simulink model "pi_simulation"  (R2023b)
settings: Solver=FixedStepAuto  StartTime=0.0  StopTime=sim_time  FixedStep=T_vz  RelTol=1e-3
values from neighbouring files (symbols this model uses):
  B_e = 0.05    [GA.m]    (also in exam.m = 0.001; grafs.m = gears(i); pi_GA.m; test.m = 0.001)
  B_m = 0.000080292    (= 8.0292e-05)    [GA.m]    (also in exam.m; pi_GA.m; test.m)
  B_z = 0.00020000    (= 0.0002)    [GA.m]    (also in exam.m; pi_GA.m; test.m)
  i_gear = 100    [GA.m]    (also in grafs.m = 20; pi_GA.m; test.m = 1)
  J_m = 0.00009    (= 9e-05)    [GA.m]    (also in exam.m; pi_GA.m; test.m)
  J_z = 0.00024943    [GA.m]    (also in exam.m; pi_GA.m; test.m)
  K_e = 0.5    [GA.m]    (also in exam.m = 0.01; grafs.m = gears(i); pi_GA.m; test.m = 0.01)
  Kd = 0.001    [test.m]
  Ki = 1.5    [test.m]
  Kp = 5    [test.m]
  M_m = 0.108    [GA.m]    (also in exam.m; pi_GA.m; test.m)
  M_z0m = 0.0052    [GA.m]    (also in exam.m; pi_GA.m; test.m)
  M_z0z = 0.0078    [GA.m]    (also in exam.m; pi_GA.m; test.m)
  N_el = 10000    [GA.m]    (also in exam.m; pi_GA.m; test.m)
  T_n = 0.001    [GA.m]    (also in exam.m; pi_GA.m; test.m)
  T_vz = 0.001    [GA.m]    (also in exam.m; pi_GA.m; test.m)
undefined symbols (not defined in the file or in its folder): DiscIntNeverNeededParam, param
libraries: slpidlib x6, simulink x3
settings Model: Creator=laptop  LastModifiedBy=maros-pc
settings SolverCC: ConsecutiveZCsStepRelTol=100000*128*eps  EnableFixedStepZeroCrossing=on  MaxZcPerStep=5
settings HardwareCC: ProdBitPerLong=64  ProdHWDeviceType=Intel->x86-64 (Linux 64)

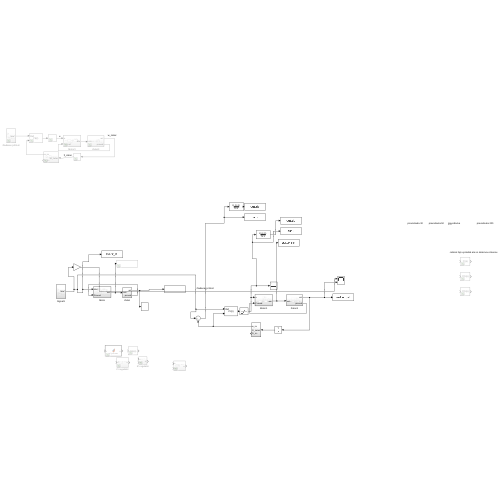
[thumbnail: Simulink's stored preview of the top-level diagram]
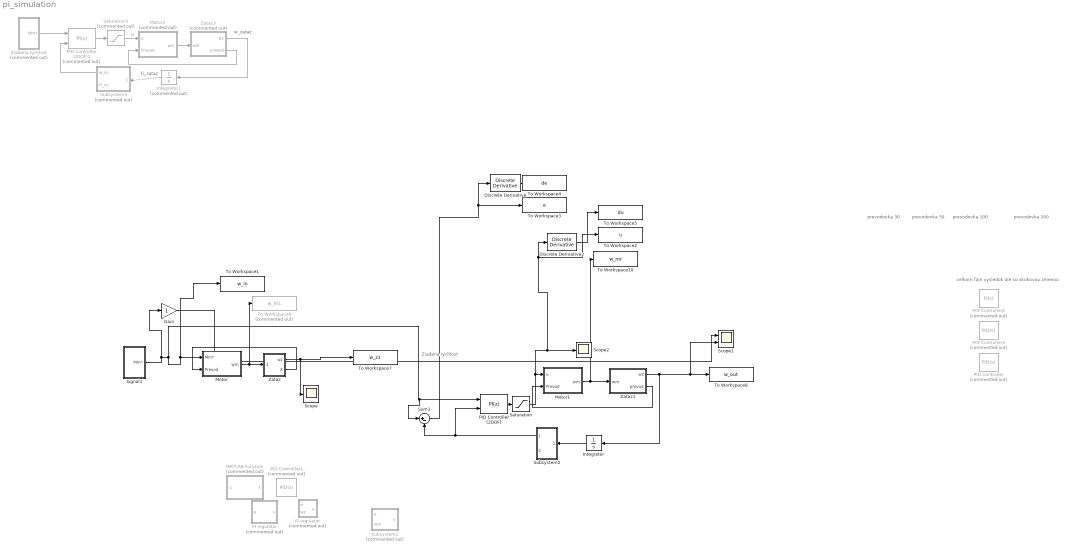
== system pi_simulation ==
  note: u
  note: w_zataz
  note: prevodovka 100
  note: celkom fajn vysledok ale so skokovou zmenou
  note: Ziadana rychlost
  note: prevodovka 200
  note: prevodovka 50
  note: prevodovka 30
  note: fi_zataz
  Discrete Derivative : simulink/Discrete/Discrete Derivative  gainval=1.0  ICPrevScaledInput=0.0  OutMin=[]  OutMax=[]  OutDataType=fixdt(1, 16)  OutScaling=2^-10  DoSatur=off
  Discrete Derivative2 : simulink/Discrete/Discrete Derivative  gainval=1.0  ICPrevScaledInput=0.0  OutMin=[]  OutMax=[]  OutDataType=fixdt(1, 16)  OutScaling=2^-10  DoSatur=off
  Gain : Gain
  IP regulator : Subsystem  Commented=on
  Integrator : Integrator
  Integrator1 : Integrator  Commented=on
  MATLAB Function : MATLAB Function  Commented=on  TreatAsAtomicUnit=on
  Motor : Subsystem
  Motor1 : Subsystem
  Motor3 : Subsystem  Commented=on
  PI regulator : Subsystem  Commented=on
  PID Controller : slpidlib/PID Controller  Commented=on  Controller=PID  Form=Parallel  TimeDomain=Continuous-time  UseExternalTs=off  SampleTime=-1  IntegratorMethod=Forward Euler  FilterMethod=Forward Euler  ControllerParametersSource=internal  P=param(1)  I=param(2)  UseKiTs=off  D=param(3)  N=param(4)  UseFilter=on  TunerSelectOption=Transfer Function Based (PID Tuner App)  InitialConditionSource=internal  InitialConditionForIntegrator=0  InitialConditionForFilter=0  DifferentiatorICPrevScaledInput=0  ExternalReset=none  TrackingMode=off  Kt=1  LimitOutput=off  SatLimitsSource=internal  UpperSaturationLimit=inf  LowerSaturationLimit=-inf  LinearizeAsGain=on  AntiWindupMode=none  Kb=1  LimitIntegrator=off  UpperIntegratorSaturationLimit=inf  LowerIntegratorSaturationLimit=-inf  POutMin=[]  POutMax=[]  IOutMin=[]  IOutMax=[]  DOutMin=[]  DOutMax=[]  NOutMin=[]  NOutMax=[]  SumOutMin=[]  SumOutMax=[]  SaturationOutMin=[]  SaturationOutMax=[]  PParamMin=[]  PParamMax=[]  IParamMin=[]  IParamMax=[]  DParamMin=[]  DParamMax=[]  NParamMin=[]  NParamMax=[]  KbParamMin=[]  KbParamMax=[]  KtParamMin=[]  KtParamMax=[]  KbOutMin=[]  KbOutMax=[]  KtOutMin=[]  KtOutMax=[]  IntegratorOutMin=[]  IntegratorOutMax=[]  FilterOutMin=[]  FilterOutMax=[]  SumI1OutMin=[]  SumI1OutMax=[]  SumI2OutMin=[]  SumI2OutMax=[]  SumI3OutMin=[]  SumI3OutMax=[]  SumI4OutMin=[]  SumI4OutMax=[]  SumDOutMin=[]  SumDOutMax=[]  DifferentiatorOutMin=[]  DifferentiatorOutMax=[]  FilterDiffOutCoefMin=[]  FilterDiffOutCoefMax=[]  ReciprocalOutMin=[]  ReciprocalOutMax=[]  SumDenOutMin=[]  SumDenOutMax=[]  SumNumOutMin=[]  SumNumOutMax=[]  DivideOutMin=[]  DivideOutMax=[]  UdiffTsProdOutMin=[]  UdiffTsProdOutMax=[]  NTsProdOutMin=[]  NTsProdOutMax=[]  UintegralTsProdOutMin=[]  UintegralTsProdOutMax=[]  UngainTsProdOutMin=[]  UngainTsProdOutMax=[]  ClampingZeroOutDataTypeStr=Inherit: Inherit via back propagation  ClampingZeroOutMin=[]  ClampingZeroOutMax=[]  FilterDenConstantOutDataTypeStr=Inherit: Inherit via back propagation  FilterDenConstantOutMin=[]  FilterDenConstantOutMax=[]  PCopyOutDataTypeStr=Inherit: Inherit via back propagation  PCopyOutMin=[]  PCopyOutMax=[]  NCopyOutDataTypeStr=Inherit: Inherit via back propagation  NCopyOutMin=[]  NCopyOutMax=[]  IntegratorContinuousStateAttributes=''  IntegratorStateMustResolveToSignalObject=off  IntegratorRTWStateStorageClass=Auto  FilterContinuousStateAttributes=''  FilterStateMustResolveToSignalObject=off  FilterRTWStateStorageClass=Auto  ParallelPVariant=InternalParameters  IdealPVariant=Disabled  IVariant=InternalParameters  DVariant=InternalParameters  IntegratorVariant=Continuous  SatVariant=Disabled  AWVariant=Passthrough  PCopyVariant=Disabled  TRVariant=Disabled  FdbkBlocksVariant=Forward  IdealPFdbkVariant=Disabled  SatFdbkVariant=Disabled  DerivativeFilterVariant=ContFilter  NVariant=InternalParameters  NCopyVariant=Disabled  FilterICVariant=InternalICsFilter  IntegratorICVariant=InternalICs  ExternalResetVariant=Disabled  TRSumVariant=Passthrough  SumFdbkVariant=Disabled  SumVariant=Sum_PID  TsampFilterVariant=InternalTs  TsampNgainVariant=Passthrough  TsampIntegralVariant=Disabled_SignalSpec  ExternalSaturationOutDataTypeStr=Inherit: Same as second input
  PID Controller (2DOF) : slpidlib/PID Controller (2DOF)  Controller=PI  Form=Parallel  TimeDomain=Discrete-time  UseExternalTs=off  SampleTime=T_vz  IntegratorMethod=Forward Euler  FilterMethod=Forward Euler  ControllerParametersSource=internal  P=param(1)  I=param(2)  UseKiTs=off  D=param(3)  N=param(4)  UseFilter=on  b=param(3)  c=param(6)  TunerSelectOption=Transfer Function Based (PID Tuner App)  InitialConditionSource=internal  InitialConditionForIntegrator=0  InitialConditionForFilter=0  DifferentiatorICPrevScaledInput=0  ExternalReset=none  TrackingMode=off  Kt=1  LimitOutput=off  SatLimitsSource=internal  UpperSaturationLimit=inf  LowerSaturationLimit=-inf  LinearizeAsGain=on  AntiWindupMode=none  Kb=1  LimitIntegrator=off  UpperIntegratorSaturationLimit=inf  LowerIntegratorSaturationLimit=-inf  POutMin=[]  POutMax=[]  IOutMin=[]  IOutMax=[]  DOutMin=[]  DOutMax=[]  NOutMin=[]  NOutMax=[]  bOutMin=[]  bOutMax=[]  cOutMin=[]  cOutMax=[]  SumOutMin=[]  SumOutMax=[]  SaturationOutMin=[]  SaturationOutMax=[]  PParamMin=[]  PParamMax=[]  IParamMin=[]  IParamMax=[]  DParamMin=[]  DParamMax=[]  NParamMin=[]  NParamMax=[]  bParamMin=[]  bParamMax=[]  cParamMin=[]  cParamMax=[]  KbParamMin=[]  KbParamMax=[]  KtParamMin=[]  KtParamMax=[]  KbOutMin=[]  KbOutMax=[]  KtOutMin=[]  KtOutMax=[]  IntegratorOutMin=[]  IntegratorOutMax=[]  FilterOutMin=[]  FilterOutMax=[]  SumI1OutMin=[]  SumI1OutMax=[]  SumI2OutMin=[]  SumI2OutMax=[]  SumI3OutMin=[]  SumI3OutMax=[]  SumI4OutMin=[]  SumI4OutMax=[]  SumDOutMin=[]  SumDOutMax=[]  Sum1OutMin=[]  Sum1OutMax=[]  Sum2OutMin=[]  Sum2OutMax=[]  Sum3OutMin=[]  Sum3OutMax=[]  DifferentiatorOutMin=[]  DifferentiatorOutMax=[]  FilterDiffOutCoefMin=[]  FilterDiffOutCoefMax=[]  ReciprocalOutMin=[]  ReciprocalOutMax=[]  SumDenOutMin=[]  SumDenOutMax=[]  SumNumOutMin=[]  SumNumOutMax=[]  DivideOutMin=[]  DivideOutMax=[]  UdiffTsProdOutMin=[]  UdiffTsProdOutMax=[]  NTsProdOutMin=[]  NTsProdOutMax=[]  UintegralTsProdOutMin=[]  UintegralTsProdOutMax=[]  UngainTsProdOutMin=[]  UngainTsProdOutMax=[]  ClampingZeroOutDataTypeStr=Inherit: Inherit via back propagation  ClampingZeroOutMin=[]  ClampingZeroOutMax=[]  FilterDenConstantOutDataTypeStr=Inherit: Inherit via back propagation  FilterDenConstantOutMin=[]  FilterDenConstantOutMax=[]  PCopyOutDataTypeStr=Inherit: Inherit via back propagation  PCopyOutMin=[]  PCopyOutMax=[]  NCopyOutDataTypeStr=Inherit: Inherit via back propagation  NCopyOutMin=[]  NCopyOutMax=[]  IntegratorContinuousStateAttributes=''  IntegratorStateMustResolveToSignalObject=off  IntegratorRTWStateStorageClass=Auto  FilterContinuousStateAttributes=''  FilterStateMustResolveToSignalObject=off  FilterRTWStateStorageClass=Auto  ParallelPVariant=InternalParameters  IdealPVariant=Disabled  IVariant=InternalParameters  DVariant=Disabled  bVariant=InternalParameters  cVariant=Disabled  IntegratorVariant=Discrete  SatVariant=Disabled  AWVariant=Passthrough  PCopyVariant=Disabled  TRVariant=Disabled  FdbkBlocksVariant=Forward  IdealPFdbkVariant=Disabled  SatFdbkVariant=Disabled  DerivativeFilterVariant=Disabled  NVariant=Disabled  NCopyVariant=Disabled_SignalSpec  FilterICVariant=Disabled  IntegratorICVariant=InternalICs  ExternalResetVariant=Disabled  TRSumVariant=Passthrough  SumFdbkVariant=Disabled  SumVariant=Sum_PI  TsampFilterVariant=InternalTs  TsampNgainVariant=Passthrough  TsampIntegralVariant=Disabled_SignalSpec  ExternalSaturationOutDataTypeStr=Inherit: Same as second input
  PID Controller (2DOF)1 : slpidlib/PID Controller (2DOF)  Commented=on  Controller=PI  Form=Parallel  TimeDomain=Discrete-time  UseExternalTs=off  SampleTime=T_vz  IntegratorMethod=Forward Euler  FilterMethod=Forward Euler  ControllerParametersSource=internal  P=param(1)  I=param(2)  UseKiTs=off  D=param(3)  N=param(4)  UseFilter=on  b=param(3)  c=param(6)  TunerSelectOption=Transfer Function Based (PID Tuner App)  InitialConditionSource=internal  InitialConditionForIntegrator=0  InitialConditionForFilter=0  DifferentiatorICPrevScaledInput=0  ExternalReset=none  TrackingMode=off  Kt=1  LimitOutput=off  SatLimitsSource=internal  UpperSaturationLimit=inf  LowerSaturationLimit=-inf  LinearizeAsGain=on  AntiWindupMode=none  Kb=1  LimitIntegrator=off  UpperIntegratorSaturationLimit=inf  LowerIntegratorSaturationLimit=-inf  POutMin=[]  POutMax=[]  IOutMin=[]  IOutMax=[]  DOutMin=[]  DOutMax=[]  NOutMin=[]  NOutMax=[]  bOutMin=[]  bOutMax=[]  cOutMin=[]  cOutMax=[]  SumOutMin=[]  SumOutMax=[]  SaturationOutMin=[]  SaturationOutMax=[]  PParamMin=[]  PParamMax=[]  IParamMin=[]  IParamMax=[]  DParamMin=[]  DParamMax=[]  NParamMin=[]  NParamMax=[]  bParamMin=[]  bParamMax=[]  cParamMin=[]  cParamMax=[]  KbParamMin=[]  KbParamMax=[]  KtParamMin=[]  KtParamMax=[]  KbOutMin=[]  KbOutMax=[]  KtOutMin=[]  KtOutMax=[]  IntegratorOutMin=[]  IntegratorOutMax=[]  FilterOutMin=[]  FilterOutMax=[]  SumI1OutMin=[]  SumI1OutMax=[]  SumI2OutMin=[]  SumI2OutMax=[]  SumI3OutMin=[]  SumI3OutMax=[]  SumI4OutMin=[]  SumI4OutMax=[]  SumDOutMin=[]  SumDOutMax=[]  Sum1OutMin=[]  Sum1OutMax=[]  Sum2OutMin=[]  Sum2OutMax=[]  Sum3OutMin=[]  Sum3OutMax=[]  DifferentiatorOutMin=[]  DifferentiatorOutMax=[]  FilterDiffOutCoefMin=[]  FilterDiffOutCoefMax=[]  ReciprocalOutMin=[]  ReciprocalOutMax=[]  SumDenOutMin=[]  SumDenOutMax=[]  SumNumOutMin=[]  SumNumOutMax=[]  DivideOutMin=[]  DivideOutMax=[]  UdiffTsProdOutMin=[]  UdiffTsProdOutMax=[]  NTsProdOutMin=[]  NTsProdOutMax=[]  UintegralTsProdOutMin=[]  UintegralTsProdOutMax=[]  UngainTsProdOutMin=[]  UngainTsProdOutMax=[]  ClampingZeroOutDataTypeStr=Inherit: Inherit via back propagation  ClampingZeroOutMin=[]  ClampingZeroOutMax=[]  FilterDenConstantOutDataTypeStr=Inherit: Inherit via back propagation  FilterDenConstantOutMin=[]  FilterDenConstantOutMax=[]  PCopyOutDataTypeStr=Inherit: Inherit via back propagation  PCopyOutMin=[]  PCopyOutMax=[]  NCopyOutDataTypeStr=Inherit: Inherit via back propagation  NCopyOutMin=[]  NCopyOutMax=[]  IntegratorContinuousStateAttributes=''  IntegratorStateMustResolveToSignalObject=off  IntegratorRTWStateStorageClass=Auto  FilterContinuousStateAttributes=''  FilterStateMustResolveToSignalObject=off  FilterRTWStateStorageClass=Auto  ParallelPVariant=InternalParameters  IdealPVariant=Disabled  IVariant=InternalParameters  DVariant=Disabled  bVariant=InternalParameters  cVariant=Disabled  IntegratorVariant=Discrete  SatVariant=Disabled  AWVariant=Passthrough  PCopyVariant=Disabled  TRVariant=Disabled  FdbkBlocksVariant=Forward  IdealPFdbkVariant=Disabled  SatFdbkVariant=Disabled  DerivativeFilterVariant=Disabled  NVariant=Disabled  NCopyVariant=Disabled_SignalSpec  FilterICVariant=Disabled  IntegratorICVariant=InternalICs  ExternalResetVariant=Disabled  TRSumVariant=Passthrough  SumFdbkVariant=Disabled  SumVariant=Sum_PI  TsampFilterVariant=InternalTs  TsampNgainVariant=Passthrough  TsampIntegralVariant=Disabled_SignalSpec  ExternalSaturationOutDataTypeStr=Inherit: Same as second input
  PID Controller1 : slpidlib/PID Controller  Commented=on  Controller=PID  Form=Parallel  TimeDomain=Continuous-time  UseExternalTs=off  SampleTime=-1  IntegratorMethod=Forward Euler  FilterMethod=Forward Euler  ControllerParametersSource=internal  P=0.00289759486685387  I=0.00379715777918526  UseKiTs=off  D=-0.00216183829362266  N=1.34033839413506  UseFilter=on  TunerSelectOption=Transfer Function Based (PID Tuner App)  InitialConditionSource=internal  InitialConditionForIntegrator=0  InitialConditionForFilter=0  DifferentiatorICPrevScaledInput=0  ExternalReset=none  TrackingMode=off  Kt=1  LimitOutput=off  SatLimitsSource=internal  UpperSaturationLimit=inf  LowerSaturationLimit=-inf  LinearizeAsGain=on  AntiWindupMode=none  Kb=1  LimitIntegrator=off  UpperIntegratorSaturationLimit=inf  LowerIntegratorSaturationLimit=-inf  POutMin=[]  POutMax=[]  IOutMin=[]  IOutMax=[]  DOutMin=[]  DOutMax=[]  NOutMin=[]  NOutMax=[]  SumOutMin=[]  SumOutMax=[]  SaturationOutMin=[]  SaturationOutMax=[]  PParamMin=[]  PParamMax=[]  IParamMin=[]  IParamMax=[]  DParamMin=[]  DParamMax=[]  NParamMin=[]  NParamMax=[]  KbParamMin=[]  KbParamMax=[]  KtParamMin=[]  KtParamMax=[]  KbOutMin=[]  KbOutMax=[]  KtOutMin=[]  KtOutMax=[]  IntegratorOutMin=[]  IntegratorOutMax=[]  FilterOutMin=[]  FilterOutMax=[]  SumI1OutMin=[]  SumI1OutMax=[]  SumI2OutMin=[]  SumI2OutMax=[]  SumI3OutMin=[]  SumI3OutMax=[]  SumI4OutMin=[]  SumI4OutMax=[]  SumDOutMin=[]  SumDOutMax=[]  DifferentiatorOutMin=[]  DifferentiatorOutMax=[]  FilterDiffOutCoefMin=[]  FilterDiffOutCoefMax=[]  ReciprocalOutMin=[]  ReciprocalOutMax=[]  SumDenOutMin=[]  SumDenOutMax=[]  SumNumOutMin=[]  SumNumOutMax=[]  DivideOutMin=[]  DivideOutMax=[]  UdiffTsProdOutMin=[]  UdiffTsProdOutMax=[]  NTsProdOutMin=[]  NTsProdOutMax=[]  UintegralTsProdOutMin=[]  UintegralTsProdOutMax=[]  UngainTsProdOutMin=[]  UngainTsProdOutMax=[]  ClampingZeroOutDataTypeStr=Inherit: Inherit via back propagation  ClampingZeroOutMin=[]  ClampingZeroOutMax=[]  FilterDenConstantOutDataTypeStr=Inherit: Inherit via back propagation  FilterDenConstantOutMin=[]  FilterDenConstantOutMax=[]  PCopyOutDataTypeStr=Inherit: Inherit via back propagation  PCopyOutMin=[]  PCopyOutMax=[]  NCopyOutDataTypeStr=Inherit: Inherit via back propagation  NCopyOutMin=[]  NCopyOutMax=[]  IntegratorContinuousStateAttributes=''  IntegratorStateMustResolveToSignalObject=off  IntegratorRTWStateStorageClass=Auto  FilterContinuousStateAttributes=''  FilterStateMustResolveToSignalObject=off  FilterRTWStateStorageClass=Auto  ParallelPVariant=InternalParameters  IdealPVariant=Disabled  IVariant=InternalParameters  DVariant=InternalParameters  IntegratorVariant=Continuous  SatVariant=Disabled  AWVariant=Passthrough  PCopyVariant=Disabled  TRVariant=Disabled  FdbkBlocksVariant=Forward  IdealPFdbkVariant=Disabled  SatFdbkVariant=Disabled  DerivativeFilterVariant=ContFilter  NVariant=InternalParameters  NCopyVariant=Disabled  FilterICVariant=InternalICsFilter  IntegratorICVariant=InternalICs  ExternalResetVariant=Disabled  TRSumVariant=Passthrough  SumFdbkVariant=Disabled  SumVariant=Sum_PID  TsampFilterVariant=InternalTs  TsampNgainVariant=Passthrough  TsampIntegralVariant=Disabled_SignalSpec  ExternalSaturationOutDataTypeStr=Inherit: Same as second input
  PID Controller2 : slpidlib/PID Controller  Commented=on  Controller=PI  Form=Parallel  TimeDomain=Continuous-time  UseExternalTs=off  SampleTime=-1  IntegratorMethod=Forward Euler  FilterMethod=Forward Euler  ControllerParametersSource=internal  P=0.0039717054355857  I=0.00555616938335056  UseKiTs=off  D=0  N=100  UseFilter=on  TunerSelectOption=Transfer Function Based (PID Tuner App)  InitialConditionSource=internal  InitialConditionForIntegrator=0  InitialConditionForFilter=0  DifferentiatorICPrevScaledInput=0  ExternalReset=none  TrackingMode=off  Kt=1  LimitOutput=off  SatLimitsSource=internal  UpperSaturationLimit=inf  LowerSaturationLimit=-inf  LinearizeAsGain=on  AntiWindupMode=none  Kb=1  LimitIntegrator=off  UpperIntegratorSaturationLimit=inf  LowerIntegratorSaturationLimit=-inf  POutMin=[]  POutMax=[]  IOutMin=[]  IOutMax=[]  DOutMin=[]  DOutMax=[]  NOutMin=[]  NOutMax=[]  SumOutMin=[]  SumOutMax=[]  SaturationOutMin=[]  SaturationOutMax=[]  PParamMin=[]  PParamMax=[]  IParamMin=[]  IParamMax=[]  DParamMin=[]  DParamMax=[]  NParamMin=[]  NParamMax=[]  KbParamMin=[]  KbParamMax=[]  KtParamMin=[]  KtParamMax=[]  KbOutMin=[]  KbOutMax=[]  KtOutMin=[]  KtOutMax=[]  IntegratorOutMin=[]  IntegratorOutMax=[]  FilterOutMin=[]  FilterOutMax=[]  SumI1OutMin=[]  SumI1OutMax=[]  SumI2OutMin=[]  SumI2OutMax=[]  SumI3OutMin=[]  SumI3OutMax=[]  SumI4OutMin=[]  SumI4OutMax=[]  SumDOutMin=[]  SumDOutMax=[]  DifferentiatorOutMin=[]  DifferentiatorOutMax=[]  FilterDiffOutCoefMin=[]  FilterDiffOutCoefMax=[]  ReciprocalOutMin=[]  ReciprocalOutMax=[]  SumDenOutMin=[]  SumDenOutMax=[]  SumNumOutMin=[]  SumNumOutMax=[]  DivideOutMin=[]  DivideOutMax=[]  UdiffTsProdOutMin=[]  UdiffTsProdOutMax=[]  NTsProdOutMin=[]  NTsProdOutMax=[]  UintegralTsProdOutMin=[]  UintegralTsProdOutMax=[]  UngainTsProdOutMin=[]  UngainTsProdOutMax=[]  ClampingZeroOutDataTypeStr=Inherit: Inherit via back propagation  ClampingZeroOutMin=[]  ClampingZeroOutMax=[]  FilterDenConstantOutDataTypeStr=Inherit: Inherit via back propagation  FilterDenConstantOutMin=[]  FilterDenConstantOutMax=[]  PCopyOutDataTypeStr=Inherit: Inherit via back propagation  PCopyOutMin=[]  PCopyOutMax=[]  NCopyOutDataTypeStr=Inherit: Inherit via back propagation  NCopyOutMin=[]  NCopyOutMax=[]  IntegratorContinuousStateAttributes=''  IntegratorStateMustResolveToSignalObject=off  IntegratorRTWStateStorageClass=Auto  FilterContinuousStateAttributes=''  FilterStateMustResolveToSignalObject=off  FilterRTWStateStorageClass=Auto  ParallelPVariant=InternalParameters  IdealPVariant=Disabled  IVariant=InternalParameters  DVariant=Disabled  IntegratorVariant=Continuous  SatVariant=Disabled  AWVariant=Passthrough  PCopyVariant=Disabled  TRVariant=Disabled  FdbkBlocksVariant=Forward  IdealPFdbkVariant=Disabled  SatFdbkVariant=Disabled  DerivativeFilterVariant=Disabled  NVariant=Disabled  NCopyVariant=Disabled_SignalSpec  FilterICVariant=Disabled  IntegratorICVariant=InternalICs  ExternalResetVariant=Disabled  TRSumVariant=Passthrough  SumFdbkVariant=Disabled  SumVariant=Sum_PI  TsampFilterVariant=InternalTs  TsampNgainVariant=Passthrough  TsampIntegralVariant=Disabled_SignalSpec  ExternalSaturationOutDataTypeStr=Inherit: Same as second input
  PID Controller3 : slpidlib/PID Controller  Commented=on  Controller=PID  Form=Parallel  TimeDomain=Continuous-time  UseExternalTs=off  SampleTime=-1  IntegratorMethod=Forward Euler  FilterMethod=Forward Euler  ControllerParametersSource=internal  P=0.00146819518976187  I=0.0028749942576144  UseKiTs=off  D=-0.001808078912925  N=0.812019419764548  UseFilter=on  TunerSelectOption=Transfer Function Based (PID Tuner App)  InitialConditionSource=internal  InitialConditionForIntegrator=0  InitialConditionForFilter=0  DifferentiatorICPrevScaledInput=0  ExternalReset=none  TrackingMode=off  Kt=1  LimitOutput=off  SatLimitsSource=internal  UpperSaturationLimit=inf  LowerSaturationLimit=-inf  LinearizeAsGain=on  AntiWindupMode=none  Kb=1  LimitIntegrator=off  UpperIntegratorSaturationLimit=inf  LowerIntegratorSaturationLimit=-inf  POutMin=[]  POutMax=[]  IOutMin=[]  IOutMax=[]  DOutMin=[]  DOutMax=[]  NOutMin=[]  NOutMax=[]  SumOutMin=[]  SumOutMax=[]  SaturationOutMin=[]  SaturationOutMax=[]  PParamMin=[]  PParamMax=[]  IParamMin=[]  IParamMax=[]  DParamMin=[]  DParamMax=[]  NParamMin=[]  NParamMax=[]  KbParamMin=[]  KbParamMax=[]  KtParamMin=[]  KtParamMax=[]  KbOutMin=[]  KbOutMax=[]  KtOutMin=[]  KtOutMax=[]  IntegratorOutMin=[]  IntegratorOutMax=[]  FilterOutMin=[]  FilterOutMax=[]  SumI1OutMin=[]  SumI1OutMax=[]  SumI2OutMin=[]  SumI2OutMax=[]  SumI3OutMin=[]  SumI3OutMax=[]  SumI4OutMin=[]  SumI4OutMax=[]  SumDOutMin=[]  SumDOutMax=[]  DifferentiatorOutMin=[]  DifferentiatorOutMax=[]  FilterDiffOutCoefMin=[]  FilterDiffOutCoefMax=[]  ReciprocalOutMin=[]  ReciprocalOutMax=[]  SumDenOutMin=[]  SumDenOutMax=[]  SumNumOutMin=[]  SumNumOutMax=[]  DivideOutMin=[]  DivideOutMax=[]  UdiffTsProdOutMin=[]  UdiffTsProdOutMax=[]  NTsProdOutMin=[]  NTsProdOutMax=[]  UintegralTsProdOutMin=[]  UintegralTsProdOutMax=[]  UngainTsProdOutMin=[]  UngainTsProdOutMax=[]  ClampingZeroOutDataTypeStr=Inherit: Inherit via back propagation  ClampingZeroOutMin=[]  ClampingZeroOutMax=[]  FilterDenConstantOutDataTypeStr=Inherit: Inherit via back propagation  FilterDenConstantOutMin=[]  FilterDenConstantOutMax=[]  PCopyOutDataTypeStr=Inherit: Inherit via back propagation  PCopyOutMin=[]  PCopyOutMax=[]  NCopyOutDataTypeStr=Inherit: Inherit via back propagation  NCopyOutMin=[]  NCopyOutMax=[]  IntegratorContinuousStateAttributes=''  IntegratorStateMustResolveToSignalObject=off  IntegratorRTWStateStorageClass=Auto  FilterContinuousStateAttributes=''  FilterStateMustResolveToSignalObject=off  FilterRTWStateStorageClass=Auto  ParallelPVariant=InternalParameters  IdealPVariant=Disabled  IVariant=InternalParameters  DVariant=InternalParameters  IntegratorVariant=Continuous  SatVariant=Disabled  AWVariant=Passthrough  PCopyVariant=Disabled  TRVariant=Disabled  FdbkBlocksVariant=Forward  IdealPFdbkVariant=Disabled  SatFdbkVariant=Disabled  DerivativeFilterVariant=ContFilter  NVariant=InternalParameters  NCopyVariant=Disabled  FilterICVariant=InternalICsFilter  IntegratorICVariant=InternalICs  ExternalResetVariant=Disabled  TRSumVariant=Passthrough  SumFdbkVariant=Disabled  SumVariant=Sum_PID  TsampFilterVariant=InternalTs  TsampNgainVariant=Passthrough  TsampIntegralVariant=Disabled_SignalSpec  ExternalSaturationOutDataTypeStr=Inherit: Same as second input
  Saturation : Saturate  UpperLimit=M_m*0.75  LowerLimit=-M_m*0.75
  Saturation1 : Saturate  Commented=on  UpperLimit=M_m*0.75  LowerLimit=-M_m*0.75
  Scope : Scope
  Scope1 : Scope  NumInputPorts=2
  Scope2 : Scope
  Signal1 : Subsystem
  Subsystem1 : Subsystem  Commented=on
  Subsystem2 : Subsystem
  Subsystem3 : Subsystem  Commented=on
  Sum1 : Sum  Inputs=|+-
  To Workspace1 : ToWorkspace  VariableName=w_in  SaveFormat=Timeseries  SampleTime=-1
  To Workspace10 : ToWorkspace  VariableName=w_mr  SaveFormat=Timeseries  SampleTime=-1
  To Workspace2 : ToWorkspace  VariableName=u  SaveFormat=Timeseries  SampleTime=-1
  To Workspace3 : ToWorkspace  VariableName=e  SaveFormat=Timeseries  SampleTime=-1
  To Workspace4 : ToWorkspace  VariableName=de  SaveFormat=Timeseries  SampleTime=-1
  To Workspace5 : ToWorkspace  VariableName=du  SaveFormat=Timeseries  SampleTime=-1
  To Workspace7 : ToWorkspace  VariableName=w_z1  SaveFormat=Timeseries  SampleTime=-1
  To Workspace8 : ToWorkspace  VariableName=w_out  SaveFormat=Timeseries  SampleTime=-1
  To Workspace9 : ToWorkspace  Commented=on  VariableName=w_m1  SaveFormat=Timeseries  SampleTime=-1
  Zataz : Subsystem
  Zataz1 : Subsystem
  Zataz3 : Subsystem  Commented=on
  "Ziadana rychlost " : Subsystem  Commented=on
  wires:
  Motor/1(wm) -> To Workspace9/1, Zataz/1(wm)
  Zataz/1(wz) -> Scope/1, To Workspace7/1
  Zataz/2(prevod) -> Motor/2(Prevod)
  Zataz1/2(prevod) -> Motor1/2(Prevod)
  Zataz1/1(wz) -> Integrator/1, Scope1/2, To Workspace8/1
  Motor1/1(wm) -> To Workspace10/1, Zataz1/1(wm)
  Integrator/1 -> Subsystem2/1(Fi_zataz)
  Subsystem2/1(w_irc) -> Sum1/2, PID Controller (2DOF)/2
  Signal1/1(Mm*) -> Gain/1, Sum1/1, PID Controller (2DOF)/1, To Workspace1/1, Motor/1(Mm*)
  Discrete Derivative/1 -> To Workspace4/1
  Discrete Derivative2/1 -> To Workspace5/1
  Sum1/1 -> Discrete Derivative/1, To Workspace3/1
  Saturation/1 -> To Workspace2/1, Discrete Derivative2/1, Scope2/1, Motor1/1(u)
  PID Controller (2DOF)/1 -> Saturation/1
  Gain/1 -> Scope1/1
  PID Controller (2DOF)1/1 -> Saturation1/1
  Motor3/1(wm) -> Zataz3/1(wm)
  Subsystem3/1(w_irc) -> PID Controller (2DOF)1/2
  Zataz3/2(prevod) -> Motor3/2(Prevod)
  Saturation1/1 -> Motor3/1(u)
  Integrator1/1 -> Subsystem3/1(Fi_zataz)
  Zataz3/1(wz) -> Integrator1/1
  "Ziadana rychlost "/1(Mm*) -> PID Controller (2DOF)1/1

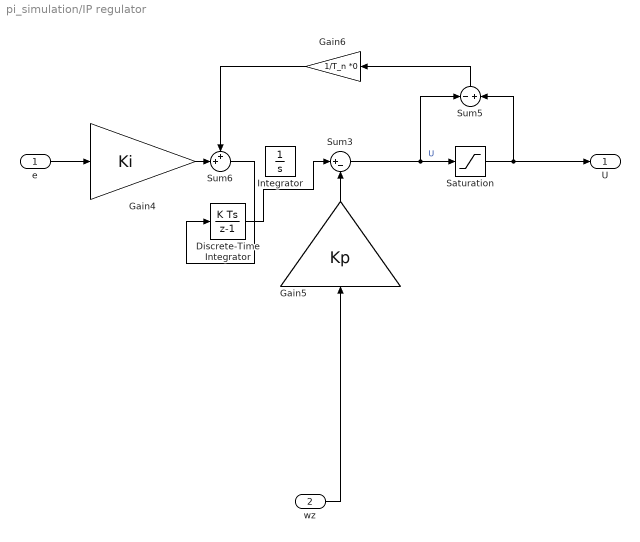
== system pi_simulation/IP regulator ==
  e : Inport
  wz : Inport  Port=2
  Discrete-Time Integrator : DiscreteIntegrator  SampleTime=-1  ICPrevOutput=DiscIntNeverNeededParam  ICPrevScaledInput=DiscIntNeverNeededParam
  Gain4 : Gain  Gain=Ki
  Gain5 : Gain  Gain=Kp
  Gain6 : Gain  Gain=1/T_n *0
  Integrator : Integrator
  Saturation : Saturate  UpperLimit=M_m*0.75  LowerLimit=-M_m*0.75
  Sum3 : Sum  Inputs=|+-
  Sum5 : Sum  Inputs=-+
  Sum6 : Sum  Inputs=++|
  U : Outport
  wires:
  Gain5/1 -> Sum3/2
  Gain4/1 -> Sum6/2
  Saturation/1 -> U/1, Sum5/2  "U"
  Sum5/1 -> Gain6/1
  Discrete-Time Integrator/1 -> Sum3/1
  Gain6/1 -> Sum6/1
  Sum3/1 -> Sum5/1, Saturation/1
  Sum6/1 -> Discrete-Time Integrator/1
  wz/1 -> Gain5/1
  e/1 -> Gain4/1

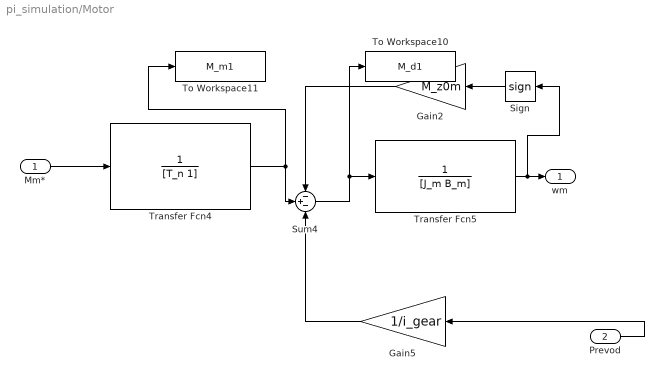
== system pi_simulation/Motor ==
  Mm* : Inport
  Prevod : Inport  Port=2
  Gain2 : Gain  Gain=M_z0m
  Gain5 : Gain  Gain=1/i_gear
  Sign : Signum
  Sum4 : Sum  Inputs=-+-
  To Workspace10 : ToWorkspace  VariableName=M_d1  SaveFormat=Timeseries  SampleTime=-1
  To Workspace11 : ToWorkspace  VariableName=M_m1  SaveFormat=Timeseries  SampleTime=-1
  Transfer Fcn4 : TransferFcn  Denominator=[T_n 1]
  Transfer Fcn5 : TransferFcn  Denominator=[J_m B_m]
  wm : Outport
  wires:
  Gain5/1 -> Sum4/3
  Sum4/1 -> To Workspace10/1, Transfer Fcn5/1
  Transfer Fcn4/1 -> Sum4/2, To Workspace11/1
  Mm*/1 -> Transfer Fcn4/1
  Prevod/1 -> Gain5/1
  Sign/1 -> Gain2/1
  Gain2/1 -> Sum4/1
  Transfer Fcn5/1 -> Sign/1, wm/1

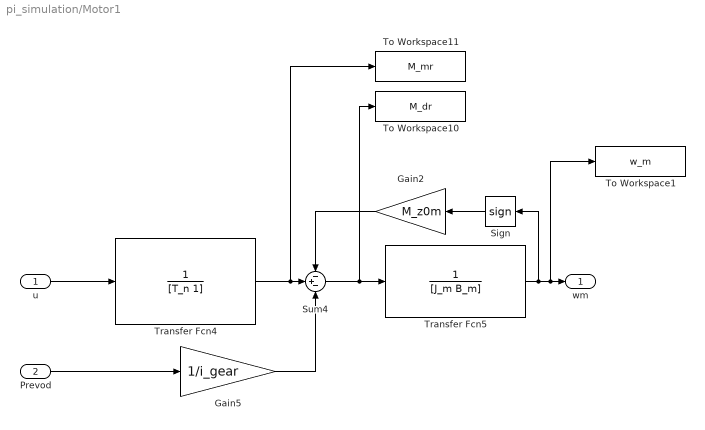
== system pi_simulation/Motor1 ==
  u : Inport
  Prevod : Inport  Port=2
  Gain2 : Gain  Gain=M_z0m
  Gain5 : Gain  Gain=1/i_gear
  Sign : Signum
  Sum4 : Sum  Inputs=-+-
  To Workspace1 : ToWorkspace  VariableName=w_m  SaveFormat=Timeseries  SampleTime=-1
  To Workspace10 : ToWorkspace  VariableName=M_dr  SaveFormat=Timeseries  SampleTime=-1
  To Workspace11 : ToWorkspace  VariableName=M_mr  SaveFormat=Timeseries  SampleTime=-1
  Transfer Fcn4 : TransferFcn  Denominator=[T_n 1]
  Transfer Fcn5 : TransferFcn  Denominator=[J_m B_m]
  wm : Outport
  wires:
  Gain5/1 -> Sum4/3
  Sum4/1 -> To Workspace10/1, Transfer Fcn5/1
  Transfer Fcn4/1 -> To Workspace11/1, Sum4/2
  u/1 -> Transfer Fcn4/1
  Prevod/1 -> Gain5/1
  Gain2/1 -> Sum4/1
  Transfer Fcn5/1 -> Sign/1, To Workspace1/1, wm/1
  Sign/1 -> Gain2/1

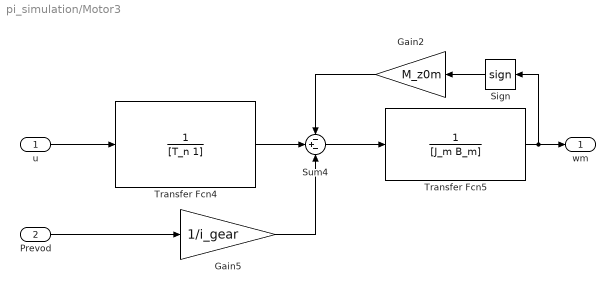
== system pi_simulation/Motor3 ==
  u : Inport
  Prevod : Inport  Port=2
  Gain2 : Gain  Gain=M_z0m
  Gain5 : Gain  Gain=1/i_gear
  Sign : Signum
  Sum4 : Sum  Inputs=-+-
  Transfer Fcn4 : TransferFcn  Denominator=[T_n 1]
  Transfer Fcn5 : TransferFcn  Denominator=[J_m B_m]
  wm : Outport
  wires:
  Gain5/1 -> Sum4/3
  Sum4/1 -> Transfer Fcn5/1
  Transfer Fcn4/1 -> Sum4/2
  u/1 -> Transfer Fcn4/1
  Prevod/1 -> Gain5/1
  Gain2/1 -> Sum4/1
  Transfer Fcn5/1 -> Sign/1, wm/1
  Sign/1 -> Gain2/1

== system pi_simulation/PI regulator ==
  e : Inport
  Discrete-Time Integrator : DiscreteIntegrator  SampleTime=T_vz  ICPrevOutput=DiscIntNeverNeededParam  ICPrevScaledInput=DiscIntNeverNeededParam
  Gain1 : Gain  Gain=Kp
  Gain2 : Gain  Gain=Ki
  Saturation : Saturate  UpperLimit=M_m*0.75  LowerLimit=-M_m*0.75
  Sum1 : Sum  Inputs=|++
  u : Outport
  wires:
  Gain1/1 -> Sum1/1
  Discrete-Time Integrator/1 -> Sum1/2
  Sum1/1 -> Saturation/1
  Gain2/1 -> Discrete-Time Integrator/1
  e/1 -> Gain2/1, Gain1/1
  Saturation/1 -> u/1  "U"

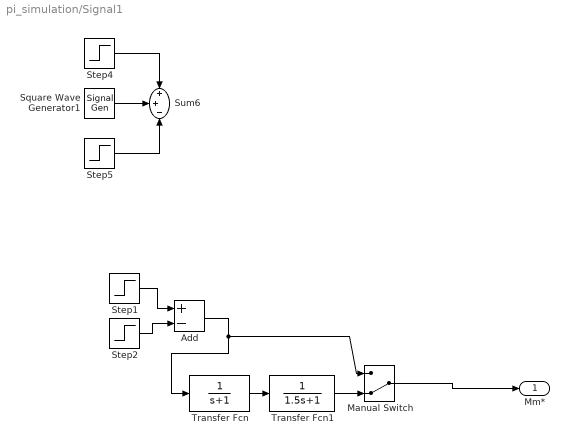
== system pi_simulation/Signal1 ==
  Add : Sum  Inputs=+-
  Manual Switch : ManualSwitch  CurrentSetting=0
  Square Wave Generator1 : SignalGenerator  Amplitude=0.8  Frequency=2
  Step1 : Step  After=pi/2  SampleTime=0
  Step2 : Step  Time=10  After=pi/2  SampleTime=0
  Step4 : Step  SampleTime=0
  Step5 : Step  Time=2  SampleTime=0
  Sum6 : Sum  Inputs=++-
  Transfer Fcn : TransferFcn  Denominator=[1 1]
  Transfer Fcn1 : TransferFcn  Denominator=[1.5 1]
  Mm* : Outport
  wires:
  Step4/1 -> Sum6/1
  Square Wave Generator1/1 -> Sum6/2
  Step5/1 -> Sum6/3
  Step1/1 -> Add/1
  Step2/1 -> Add/2
  Transfer Fcn/1 -> Transfer Fcn1/1
  Transfer Fcn1/1 -> Manual Switch/2
  Manual Switch/1 -> Mm*/1
  Add/1 -> Manual Switch/1, Transfer Fcn/1

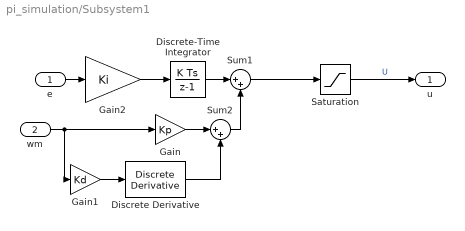
== system pi_simulation/Subsystem1 ==
  e : Inport
  wm : Inport  Port=2
  Discrete Derivative : simulink/Discrete/Discrete Derivative  gainval=1.0  ICPrevScaledInput=0.0  OutMin=[]  OutMax=[]  OutDataType=fixdt(1, 16)  OutScaling=2^-10  DoSatur=off
  Discrete-Time Integrator : DiscreteIntegrator  SampleTime=T_vz  ICPrevOutput=DiscIntNeverNeededParam  ICPrevScaledInput=DiscIntNeverNeededParam
  Gain : Gain  Gain=Kp
  Gain1 : Gain  Gain=Kd
  Gain2 : Gain  Gain=Ki
  Saturation : Saturate  UpperLimit=M_m*0.75  LowerLimit=-M_m*0.75
  Sum1 : Sum  Inputs=|++
  Sum2 : Sum  Inputs=|++
  u : Outport
  wires:
  Discrete-Time Integrator/1 -> Sum1/1
  Sum1/1 -> Saturation/1
  Gain2/1 -> Discrete-Time Integrator/1
  e/1 -> Gain2/1
  Saturation/1 -> u/1  "U"
  Gain1/1 -> Discrete Derivative/1
  Gain/1 -> Sum2/1
  Discrete Derivative/1 -> Sum2/2
  Sum2/1 -> Sum1/2
  wm/1 -> Gain1/1, Gain/1

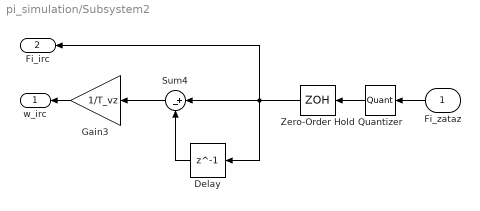
== system pi_simulation/Subsystem2 ==
  Fi_zataz : Inport
  Delay : Delay  DelayLength=1
  Gain3 : Gain  Gain=1/T_vz
  Quantizer : Quantizer  QuantizationInterval=2*pi/N_el
  Sum4 : Sum  Inputs=|+-
  Zero-Order Hold : ZeroOrderHold  SampleTime=T_vz
  w_irc : Outport
  Fi_irc : Outport  Port=2
  wires:
  Sum4/1 -> Gain3/1
  Delay/1 -> Sum4/2
  Zero-Order Hold/1 -> Delay/1, Sum4/1, Fi_irc/1
  Fi_zataz/1 -> Quantizer/1
  Quantizer/1 -> Zero-Order Hold/1
  Gain3/1 -> w_irc/1

== system pi_simulation/Subsystem3 ==
  Fi_zataz : Inport
  Delay : Delay  DelayLength=1
  Gain3 : Gain  Gain=1/T_vz
  Quantizer : Quantizer  QuantizationInterval=2*pi/N_el
  Sum4 : Sum  Inputs=|+-
  Zero-Order Hold : ZeroOrderHold  SampleTime=T_vz
  w_irc : Outport
  Fi_irc : Outport  Port=2
  wires:
  Sum4/1 -> Gain3/1
  Delay/1 -> Sum4/2
  Zero-Order Hold/1 -> Delay/1, Sum4/1, Fi_irc/1
  Fi_zataz/1 -> Quantizer/1
  Quantizer/1 -> Zero-Order Hold/1
  Gain3/1 -> w_irc/1

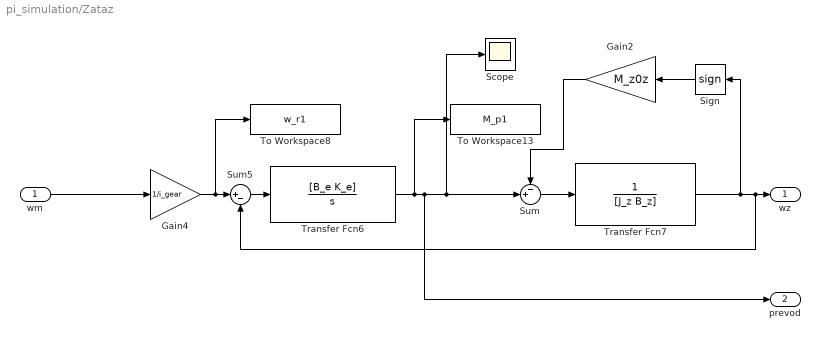
== system pi_simulation/Zataz ==
  wm : Inport
  Gain2 : Gain  Gain=M_z0z
  Gain4 : Gain  Gain=1/i_gear
  Scope : Scope
  Sign : Signum
  Sum : Sum  Inputs=-+|
  Sum5 : Sum  Inputs=|+-
  To Workspace13 : ToWorkspace  VariableName=M_p1  SaveFormat=Timeseries  SampleTime=-1
  To Workspace8 : ToWorkspace  VariableName=w_r1  SaveFormat=Timeseries  SampleTime=-1
  Transfer Fcn6 : TransferFcn  Numerator=[B_e K_e]  Denominator=[1 0]
  Transfer Fcn7 : TransferFcn  Denominator=[J_z B_z]
  wz : Outport
  prevod : Outport  Port=2
  wires:
  wm/1 -> Gain4/1
  Sum5/1 -> Transfer Fcn6/1
  Transfer Fcn6/1 -> To Workspace13/1, prevod/1, Sum/2, Scope/1
  Gain4/1 -> To Workspace8/1, Sum5/1
  Sign/1 -> Gain2/1
  Gain2/1 -> Sum/1
  Transfer Fcn7/1 -> Sign/1, Sum5/2, wz/1
  Sum/1 -> Transfer Fcn7/1

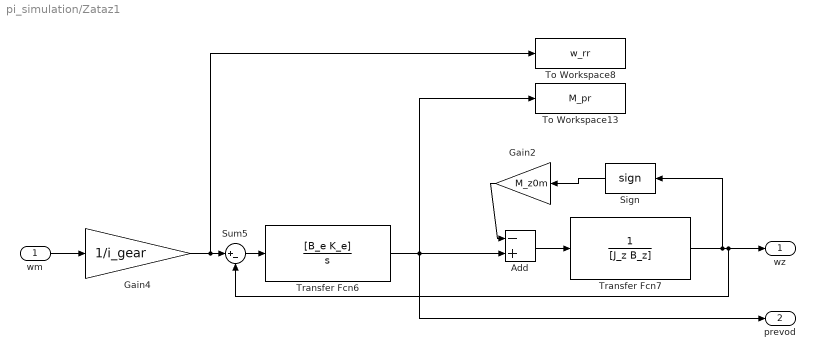
== system pi_simulation/Zataz1 ==
  wm : Inport
  Add : Sum  Inputs=-+
  Gain2 : Gain  Gain=M_z0m
  Gain4 : Gain  Gain=1/i_gear
  Sign : Signum
  Sum5 : Sum  Inputs=|+-
  To Workspace13 : ToWorkspace  VariableName=M_pr  SaveFormat=Timeseries  SampleTime=-1
  To Workspace8 : ToWorkspace  VariableName=w_rr  SaveFormat=Timeseries  SampleTime=-1
  Transfer Fcn6 : TransferFcn  Numerator=[B_e K_e]  Denominator=[1 0]
  Transfer Fcn7 : TransferFcn  Denominator=[J_z B_z]
  wz : Outport
  prevod : Outport  Port=2
  wires:
  wm/1 -> Gain4/1
  Sum5/1 -> Transfer Fcn6/1
  Transfer Fcn6/1 -> To Workspace13/1, Add/2, prevod/1
  Gain4/1 -> To Workspace8/1, Sum5/1
  Transfer Fcn7/1 -> Sign/1, wz/1, Sum5/2
  Gain2/1 -> Add/1
  Add/1 -> Transfer Fcn7/1
  Sign/1 -> Gain2/1

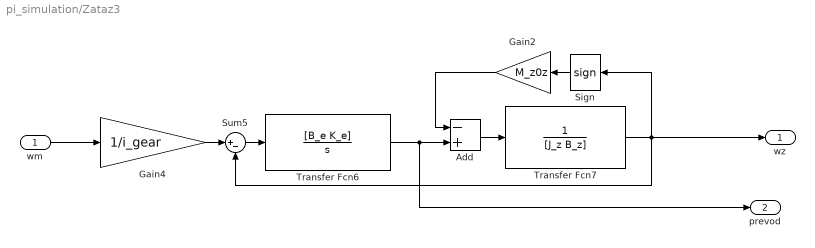
== system pi_simulation/Zataz3 ==
  wm : Inport
  Add : Sum  Inputs=-+
  Gain2 : Gain  Gain=M_z0z
  Gain4 : Gain  Gain=1/i_gear
  Sign : Signum
  Sum5 : Sum  Inputs=|+-
  Transfer Fcn6 : TransferFcn  Numerator=[B_e K_e]  Denominator=[1 0]
  Transfer Fcn7 : TransferFcn  Denominator=[J_z B_z]
  wz : Outport
  prevod : Outport  Port=2
  wires:
  wm/1 -> Gain4/1
  Sum5/1 -> Transfer Fcn6/1
  Transfer Fcn6/1 -> Add/2, prevod/1
  Gain4/1 -> Sum5/1
  Transfer Fcn7/1 -> wz/1, Sign/1, Sum5/2
  Gain2/1 -> Add/1
  Add/1 -> Transfer Fcn7/1
  Sign/1 -> Gain2/1

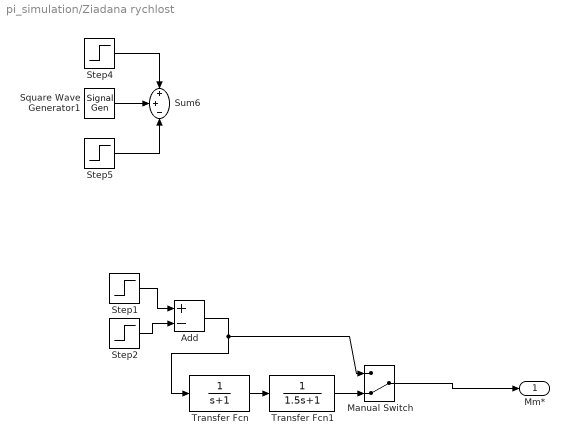
== system pi_simulation/Ziadana rychlost  ==
  Add : Sum  Inputs=+-
  Manual Switch : ManualSwitch  CurrentSetting=0
  Square Wave Generator1 : SignalGenerator  Amplitude=0.8  Frequency=2
  Step1 : Step  After=pi/2  SampleTime=0
  Step2 : Step  Time=10  After=pi/2  SampleTime=0
  Step4 : Step  SampleTime=0
  Step5 : Step  Time=2  SampleTime=0
  Sum6 : Sum  Inputs=++-
  Transfer Fcn : TransferFcn  Denominator=[1 1]
  Transfer Fcn1 : TransferFcn  Denominator=[1.5 1]
  Mm* : Outport
  wires:
  Step4/1 -> Sum6/1
  Square Wave Generator1/1 -> Sum6/2
  Step5/1 -> Sum6/3
  Step1/1 -> Add/1
  Step2/1 -> Add/2
  Transfer Fcn/1 -> Transfer Fcn1/1
  Transfer Fcn1/1 -> Manual Switch/2
  Manual Switch/1 -> Mm*/1
  Add/1 -> Manual Switch/1, Transfer Fcn/1

== matlab function pi_simulation/MATLAB Function ==
  data: u input; x output
function x = signum(u)
%SIGNUM Summary of this function goes here
%   Detailed explanation goes here
    if(u > 0)
        x = 1;
    elseif(u < 0)
        x = -1;
    else
        x = 0;
    end
end
